simulink model "Predefined_with_GroundTruth_mod22vig1"  (R2022b)
settings: Solver=ode45  StartTime=0.0  StopTime=inf  MaxStep=0.01  RelTol=1e-3
PreLoadFcn:
  | old_index = 1;
model workspace (MAT data in the model file):
  firstWarning = 1
  originalScenarioChecksum = '114339432DE22364D47BB28FC96DC10C'
undefined symbols (not defined in the file or in its folder): Acceleration, ActorID, AngularVelocity, curvature, curvatureAhd, DefaultGear, DEND_B, DEND_S, DEND_T, direction, DiscIntNeverNeededParam, driving, gradbp, L, LF, LR, matlabshared, MAX_BRAKE, MAX_STEER, MAX_TORQUE, MCAR, MIN_BRAKE, MIN_STEER, MIN_TORQUE, NUMD_B, NUMD_S, NUMD_T, Pitch, Position, psi_o, R, Roll, RRdamp, SceneInfo, session, sigbuilder_block, STEER_RATIO, stopSign_ID, Tdead, thetaRefs, TL_ID, TrackWidth, Ts, ts, Vdead, Velocity, WB, X_o, xRef2, xRef2s, Y_o, Yaw, yRef2, yRef2s
libraries: mpcsigdimcheck_private x10, drivingscenarioandsensors x8, drivingvehiclecontroller x2, eeGeneralControl x2, slpidlib x2, simulink x2, trackingutilitieslib x2, mpclib x1, mpcadaslib x1, robotalgslib x1, simulink_extras x1, drivinglib x1
(part 1 of 3)
settings Model: Creator=akshran  LastModifiedBy=rahulmathias
settings DataIOCC: SignalLogging=off
settings DebuggingCC: UnconnectedInputMsg=warning  UnconnectedOutputMsg=warning  UnconnectedLineMsg=warning
settings HardwareCC: ProdBitPerLong=64  ProdHWDeviceType=Intel->x86-64 (Mac OS X)
settings ModelReferenceCC: EnableRefExpFcnMdlSchedulingChecks=on
settings RTWCC: DLArmComputeVersion=19.05

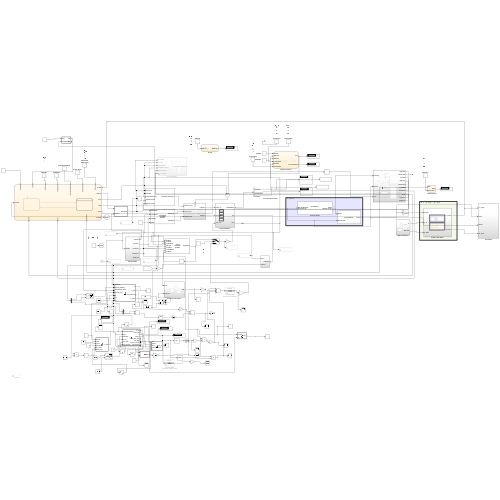
[thumbnail: Simulink's stored preview of the top-level diagram]
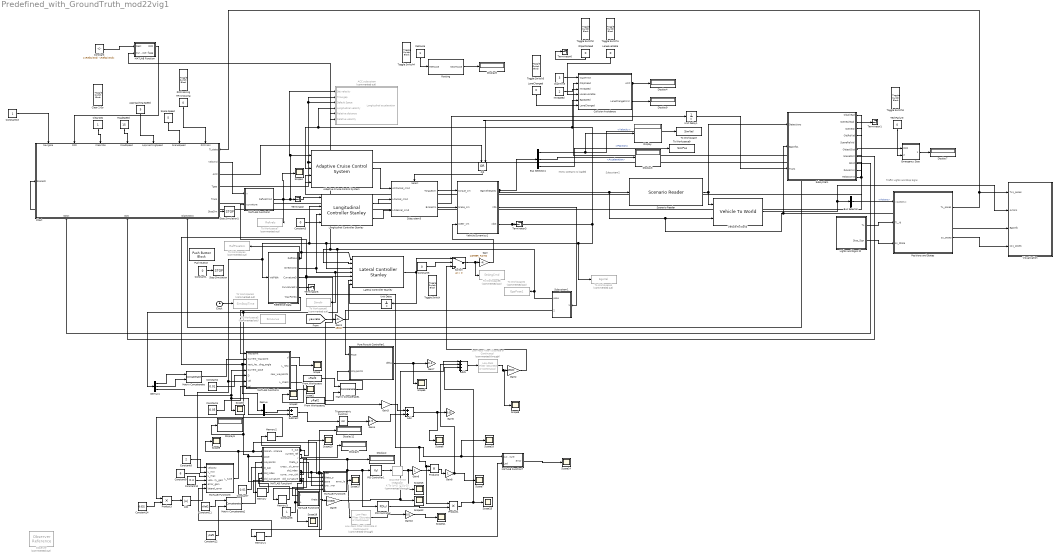
== system Predefined_with_GroundTruth_mod22vig1 ==
  note: Subsystem2
  note: Mcity scenario is loaded
  note: Traffic Lights and Stop Signs
  ACC subsystem : Subsystem  Commented=on
  Abs : Abs  SaturateOnIntegerOverflow=off
  Adaptive Cruise Control System : mpcadaslib/Adaptive Cruise Control System  EgoModel=tf(1,[0.5,1,0])  InitialEgoVelocity=0  DefaultSpacing=WB+2  MaxVelocity=50  MinAcceleration=-40  amin_ext=off  MaxAcceleration=40  amax_ext=off  Ts=0.1  PredictionHorizon=10  ControllerBehavior=1.0  suboptimal=off  maxiter=10  datatypeopt=double  optmode=off  trackmode=off
  Add : Sum
  Add1 : Sum  Inputs=++++
  Approaching Speed : Constant  Value=5
  Bus Selector : BusSelector  OutputSignals=Actors
  Bus Selector4 : BusSelector  OutputSignals=Velocity,Acceleration,Position
  Chart : Stateflow chart  TreatAsAtomicUnit=on
      settings: PortSchema="{\"entries\":[{\"content\":{\"sides\":[{\"content\":{\"connectorIds\":[\"In12\"]},\"type\":\"ConnectorPlacement.EquallySpacedRectSide\",\"uuid\":\"81aca70f-0947-49fb-b60a-be241e44193b\"},{\"content\":{\"connectorIds\":[\"In1\",\"Out1\",\"Out2\",\"Out3\",\"Out4\",\"Out5\"],\"side\":\"RIGHT\"},\"type\":\"ConnectorPlacement.EquallySpacedRectSide\",\"uuid\":\"e7b9645e-3711-4964-ac9b-0199dd335e99\"},{\"content\":{\"connectorIds\":[\"In8\",\"In9\",\"In10\",\"In11\",\"In2\",\"In4\",\"In6\"],\"side\":\"TOP\"},\"type\":\"ConnectorPlacement.EquallySpacedRectSide\",\"uuid\":\"6876f024-944b-4540-9404-d68f37763657\"},{\"content\":{\"connectorIds\":[\"In5\",\"In7\",\"In3\"],\"side\":\"BOTTOM\"},\"type\":\"ConnectorPlacement.EquallySpacedRectSide\",\"uuid\":\"44acab73-cdde-4edf-95df-27422644ccab\"}]},\"type\":\"ConnectorPlacement.EquallySpacedConnector\",\"uuid\":\"d2c31c01-e447-43db-8d2b-8b98a0ca291a\"}],\"packageUris\":[\"http://schema.mathworks.com/mf0/Connector/R2020b\"],\"version\":\"1.0\"}"
  Clear 2 Go : ToggleSwitchBlock
      settings: Values={{'Off', 'On'}, [0 1]}
  Clear2Go : Constant
  Clock : Clock
  Collision Avoidance : Stateflow chart  TreatAsAtomicUnit=on
  Constant : Constant  Value=[xRef2s(end) -yRef2s(end)]
  Constant1 : Constant  Value=0
  Constant10 : Constant  Value=0.4
  Constant11 : Constant  Value=xRef2
  Constant12 : Constant  Value=yRef2
  Constant13 : Constant
  Constant14 : Constant  Value=0.032
  Constant2 : Constant  Value=0.01
  Constant3 : Constant  Value=0
  Constant4 : Constant  Value=0.05
  Constant5 : Constant  Value=0
  Constant6 : Constant  Value=L
  Constant7 : Constant  Value=0.01
  Constant8 : Constant  Value=2
  Constant9 : Constant  Value=6
  Demux : Demux  Outputs=3
  Demux1 : Demux  Outputs=3
  Discrete-Time Integrator : DiscreteIntegrator  Commented=through  IntegratorMethod=Integration: Trapezoidal  SampleTime=-1  ICPrevOutput=DiscIntNeverNeededParam  ICPrevScaledInput=DiscIntNeverNeededParam
  Display{,2..9,12} (10 alike) : Display
  Emergency Stop : Stateflow chart  TreatAsAtomicUnit=on
  From Workspace : FromWorkspace  VariableName=xRef2
  From Workspace1 : FromWorkspace  VariableName=yRef2
  Gain : Gain  Gain=1/STEER_RATIO
  Gain1 : Gain  Gain=180/pi
  Gain10 : Gain  Gain=0.01
  Gain2 : Gain  Gain=180/pi
  Gain3 : Gain  Gain=6*6/2
  Gain4 : Gain  Gain=3.5
  Gain5 : Gain  Gain=0.05
  Gain6 : Gain
  Gain7 : Gain  Gain=0.4
  Gain8 : Gain
  Gain9 : Gain  Gain=0.5305
  LaneAvailable : Constant  Value=0
  LaneChanged : Constant  Value=0
  Lateral Controller Stanley : drivingvehiclecontroller/Lateral Controller Stanley  ModelType=Dynamic bicycle model  PositionGainF=2.5  PositionGainR=2.5  YawRateGain=0.2  DelayGain=0.2  VehicleMass=MCAR  Lf=LF  Lr=LR  TireStiffness=5e3  Wheelbase=3  MaxSteeringAngle=80
  Lights and Signs ID : Subsystem
  Longitudinal Controller Stanley : drivingvehiclecontroller/Longitudinal Controller Stanley  Kp=10  Ki=0.1  SampleTime=0.05  MaxAcceleration=40  MaxDeceleration=40
  Low-Pass Filter (Discrete or Continuous) : eeGeneralControl/Low-Pass Filter (Discrete or Continuous)  Commented=through  K=1  T=0.5  B=inf  A=-inf  init_option=Inherited from block input  x0=0  Ts=-1
  Low-Pass Filter (Discrete or Continuous)2 : eeGeneralControl/Low-Pass Filter (Discrete or Continuous)  Commented=through  K=1  T=1.2  B=inf  A=-inf  init_option=Inherited from block input  x0=0  Ts=-1
  MATLAB Function : MATLAB Function  TreatAsAtomicUnit=on
  MATLAB Function1 : MATLAB Function  TreatAsAtomicUnit=on
  MATLAB Function2 : MATLAB Function  TreatAsAtomicUnit=on
  MATLAB Function3 : MATLAB Function  TreatAsAtomicUnit=on
  MATLAB Function4 : MATLAB Function  TreatAsAtomicUnit=on
  MATLAB Function5 : MATLAB Function  TreatAsAtomicUnit=on
  MATLAB Function6 : MATLAB Function  TreatAsAtomicUnit=on
  MATLAB Function7 : MATLAB Function  TreatAsAtomicUnit=on
  Matrix Concatenate : Concatenate  Mode=Multidimensional array  ConcatenateDimension=2
  Matrix Concatenate1 : Concatenate  Mode=Multidimensional array  ConcatenateDimension=2
  Matrix Concatenate2 : Concatenate  Mode=Multidimensional array  ConcatenateDimension=2
  Memory : Memory  InitialCondition=1  LinearizeMemory=on
  Memory1 : Memory  LinearizeMemory=on
  Memory2 : Memory  LinearizeMemory=on
  Memory3 : Memory  LinearizeMemory=on
  MinSpeed : Constant  Value=2
  OR : Logic  Operator=OR  IconShape=distinctive  AllPortsSameDT=off  OutDataTypeStr=fixdt(1,16)
  ObjectAhead : Constant  Value=0
  Observer : ObserverReference  Commented=on  ObserverModelName=Predefined_with_GroundTruth_mod22_Observer1
  PID Controller : slpidlib/PID Controller  Controller=PD  Form=Parallel  TimeDomain=Discrete-time  UseExternalTs=off  SampleTime=-1  IntegratorMethod=Forward Euler  FilterMethod=Forward Euler  ControllerParametersSource=internal  P=0.0  I=1  UseKiTs=off  D=0.4616  N=100  UseFilter=on  TunerSelectOption=Transfer Function Based (PID Tuner App)  InitialConditionSource=internal  InitialConditionForIntegrator=0  InitialConditionForFilter=0  DifferentiatorICPrevScaledInput=0  ExternalReset=none  TrackingMode=off  Kt=1  LimitOutput=off  SatLimitsSource=internal  UpperSaturationLimit=inf  LowerSaturationLimit=-inf  LinearizeAsGain=on  AntiWindupMode=none  Kb=1  LimitIntegrator=off  UpperIntegratorSaturationLimit=inf  LowerIntegratorSaturationLimit=-inf  POutMin=[]  POutMax=[]  IOutMin=[]  IOutMax=[]  DOutMin=[]  DOutMax=[]  NOutMin=[]  NOutMax=[]  SumOutMin=[]  SumOutMax=[]  SaturationOutMin=[]  SaturationOutMax=[]  PParamMin=[]  PParamMax=[]  IParamMin=[]  IParamMax=[]  DParamMin=[]  DParamMax=[]  NParamMin=[]  NParamMax=[]  KbParamMin=[]  KbParamMax=[]  KtParamMin=[]  KtParamMax=[]  KbOutMin=[]  KbOutMax=[]  KtOutMin=[]  KtOutMax=[]  IntegratorOutMin=[]  IntegratorOutMax=[]  FilterOutMin=[]  FilterOutMax=[]  SumI1OutMin=[]  SumI1OutMax=[]  SumI2OutMin=[]  SumI2OutMax=[]  SumI3OutMin=[]  SumI3OutMax=[]  SumI4OutMin=[]  SumI4OutMax=[]  SumDOutMin=[]  SumDOutMax=[]  DifferentiatorOutMin=[]  DifferentiatorOutMax=[]  FilterDiffOutCoefMin=[]  FilterDiffOutCoefMax=[]  ReciprocalOutMin=[]  ReciprocalOutMax=[]  SumDenOutMin=[]  SumDenOutMax=[]  SumNumOutMin=[]  SumNumOutMax=[]  DivideOutMin=[]  DivideOutMax=[]  UdiffTsProdOutMin=[]  UdiffTsProdOutMax=[]  NTsProdOutMin=[]  NTsProdOutMax=[]  UintegralTsProdOutMin=[]  UintegralTsProdOutMax=[]  UngainTsProdOutMin=[]  UngainTsProdOutMax=[]  ClampingZeroOutDataTypeStr=Inherit: Inherit via back propagation  ClampingZeroOutMin=[]  ClampingZeroOutMax=[]  FilterDenConstantOutDataTypeStr=Inherit: Inherit via back propagation  FilterDenConstantOutMin=[]  FilterDenConstantOutMax=[]  PCopyOutDataTypeStr=Inherit: Inherit via back propagation  PCopyOutMin=[]  PCopyOutMax=[]  NCopyOutDataTypeStr=Inherit: Inherit via back propagation  NCopyOutMin=[]  NCopyOutMax=[]  IntegratorContinuousStateAttributes=''  IntegratorStateMustResolveToSignalObject=off  IntegratorRTWStateStorageClass=Auto  FilterContinuousStateAttributes=''  FilterStateMustResolveToSignalObject=off  FilterRTWStateStorageClass=Auto  ParallelPVariant=InternalParameters  IdealPVariant=Disabled  IVariant=Disabled  DVariant=InternalParameters  IntegratorVariant=Disabled  SatVariant=Disabled  AWVariant=Disabled  PCopyVariant=Disabled  TRVariant=Disabled  FdbkBlocksVariant=Forward  IdealPFdbkVariant=Disabled  SatFdbkVariant=Disabled  DerivativeFilterVariant=ForwardEulerFilter  NVariant=InternalParameters  NCopyVariant=Disabled  FilterICVariant=InternalICsFilter  IntegratorICVariant=Disabled  ExternalResetVariant=Disabled  TRSumVariant=Passthrough  SumFdbkVariant=Disabled  SumVariant=Sum_PD  TsampFilterVariant=InternalTs  TsampNgainVariant=Passthrough  TsampIntegralVariant=Disabled_SignalSpec  ExternalSaturationOutDataTypeStr=Inherit: Same as second input
  PID Controller1 : slpidlib/PID Controller  Controller=I  Form=Parallel  TimeDomain=Discrete-time  UseExternalTs=off  SampleTime=-1  IntegratorMethod=Trapezoidal  FilterMethod=Forward Euler  ControllerParametersSource=internal  P=1  I=0.0079  UseKiTs=on  D=0  N=100  UseFilter=on  TunerSelectOption=Transfer Function Based (PID Tuner App)  InitialConditionSource=internal  InitialConditionForIntegrator=0  InitialConditionForFilter=0  DifferentiatorICPrevScaledInput=0  ExternalReset=none  TrackingMode=off  Kt=1  LimitOutput=off  SatLimitsSource=internal  UpperSaturationLimit=inf  LowerSaturationLimit=-inf  LinearizeAsGain=on  AntiWindupMode=none  Kb=1  LimitIntegrator=off  UpperIntegratorSaturationLimit=inf  LowerIntegratorSaturationLimit=-inf  POutMin=[]  POutMax=[]  IOutMin=[]  IOutMax=[]  DOutMin=[]  DOutMax=[]  NOutMin=[]  NOutMax=[]  SumOutMin=[]  SumOutMax=[]  SaturationOutMin=[]  SaturationOutMax=[]  PParamMin=[]  PParamMax=[]  IParamMin=[]  IParamMax=[]  DParamMin=[]  DParamMax=[]  NParamMin=[]  NParamMax=[]  KbParamMin=[]  KbParamMax=[]  KtParamMin=[]  KtParamMax=[]  KbOutMin=[]  KbOutMax=[]  KtOutMin=[]  KtOutMax=[]  IntegratorOutMin=[]  IntegratorOutMax=[]  FilterOutMin=[]  FilterOutMax=[]  SumI1OutMin=[]  SumI1OutMax=[]  SumI2OutMin=[]  SumI2OutMax=[]  SumI3OutMin=[]  SumI3OutMax=[]  SumI4OutMin=[]  SumI4OutMax=[]  SumDOutMin=[]  SumDOutMax=[]  DifferentiatorOutMin=[]  DifferentiatorOutMax=[]  FilterDiffOutCoefMin=[]  FilterDiffOutCoefMax=[]  ReciprocalOutMin=[]  ReciprocalOutMax=[]  SumDenOutMin=[]  SumDenOutMax=[]  SumNumOutMin=[]  SumNumOutMax=[]  DivideOutMin=[]  DivideOutMax=[]  UdiffTsProdOutMin=[]  UdiffTsProdOutMax=[]  NTsProdOutMin=[]  NTsProdOutMax=[]  UintegralTsProdOutMin=[]  UintegralTsProdOutMax=[]  UngainTsProdOutMin=[]  UngainTsProdOutMax=[]  ClampingZeroOutDataTypeStr=Inherit: Inherit via back propagation  ClampingZeroOutMin=[]  ClampingZeroOutMax=[]  FilterDenConstantOutDataTypeStr=Inherit: Inherit via back propagation  FilterDenConstantOutMin=[]  FilterDenConstantOutMax=[]  PCopyOutDataTypeStr=Inherit: Inherit via back propagation  PCopyOutMin=[]  PCopyOutMax=[]  NCopyOutDataTypeStr=Inherit: Inherit via back propagation  NCopyOutMin=[]  NCopyOutMax=[]  IntegratorContinuousStateAttributes=''  IntegratorStateMustResolveToSignalObject=off  IntegratorRTWStateStorageClass=Auto  FilterContinuousStateAttributes=''  FilterStateMustResolveToSignalObject=off  FilterRTWStateStorageClass=Auto  ParallelPVariant=Disabled  IdealPVariant=Disabled  IVariant=InternalParameters  DVariant=Disabled  IntegratorVariant=Discrete  SatVariant=Disabled  AWVariant=Passthrough  PCopyVariant=Disabled  TRVariant=Disabled  FdbkBlocksVariant=Forward  IdealPFdbkVariant=Disabled  SatFdbkVariant=Disabled  DerivativeFilterVariant=Disabled  NVariant=Disabled  NCopyVariant=Disabled_SignalSpec  FilterICVariant=Disabled  IntegratorICVariant=InternalICs  ExternalResetVariant=Disabled  TRSumVariant=Passthrough  SumFdbkVariant=Disabled  SumVariant=Passthrough_I  TsampFilterVariant=InternalTs  TsampNgainVariant=Passthrough  TsampIntegralVariant=Passthrough  ExternalSaturationOutDataTypeStr=Inherit: Same as second input
  "Positions and States " : Subsystem
  Product1 : Product
  Product2 : Product
  Product3 : Product
  Pure Pursuit Controller1 : Subsystem
  Push Button : PushButtonBlock  OffValue=0.000000
  RR Crossing : Constant  Value=0
  RRCrossing : ToggleSwitchBlock
      settings: Values={{'Off', 'On'}, [0 1]}
  ReRoute : Constant
  Reference Data : Subsystem  VariantControl=Stanley
  RoadSpeed : Constant  Value=15
  Routing : Stateflow chart  TreatAsAtomicUnit=on
  Scenario Reader : drivingscenarioandsensors/Scenario Reader  ScenarioSource=From file  ScenarioFileName=/Users/vigneshsrinivasan/Downloads/ad2_y1_simulationpkg/scenarios/Roundabout.mat  ScenarioVariableName=scenario  OutputCoordinateSystem=Vehicle coordinates  EgoVehicleSource=Input port  EgoVehicleActorID=1  OrientVehiclesOnRoad=on  OutputEgoVehiclePose=on  OutputEgoVehicleState=off  SampleTime=Ts  LaneBoundaryOutput=None  LaneBoundaryDistance=0:0.5:9.5  LaneBoundaryLocation=Center of lane markings  BusNameSource=Auto  BusName=BusActors  BusNumActorsSource=Scenario  BusNumActors=100  BusName2Source=Auto  BusName2=BusLaneBoundaries  BusNumLaneBoundariesSource=Scenario  BusNumLaneBoundaries=10  BusName3Source=Auto  BusName3=BusEgoActor  BusName4Source=Auto  BusName4=BusEgoState  ShowCoordinateLabels=on  SimulateUsing=Interpreted execution
  Scene Speed : Constant  Value=5
  Scope{,1..15,17..19} (19 alike) : Scope
  Stop Simulation : Stop
  Stop Simulation1 : Stop
  Subsystem : Subsystem
  Subsystem1 : Subsystem
  Subsystem3 : Subsystem
      settings: PortSchema="{\"entries\":[{\"content\":{\"sides\":[{\"content\":{\"connectorIds\":[\"In1\",\"In2\",\"In3\"]},\"type\":\"ConnectorPlacement.EquallySpacedRectSide\",\"uuid\":\"a23b1a10-3bcb-40a0-900c-c9a3f160b173\"},{\"content\":{\"connectorIds\":[\"Out1\",\"Out2\"],\"side\":\"RIGHT\"},\"type\":\"ConnectorPlacement.EquallySpacedRectSide\",\"uuid\":\"88840b66-912f-4184-aeec-297642319416\"},{\"content\":{\"connectorIds\":[\"In4\"],\"side\":\"TOP\"},\"type\":\"ConnectorPlacement.EquallySpacedRectSide\",\"uuid\":\"37a03ca9-b065-473e-b290-3b07703c6005\"}]},\"type\":\"ConnectorPlacement.EquallySpacedConnector\",\"uuid\":\"5bfc7c71-8f7a-4cba-a168-7eeca22a2fcb\"}],\"packageUris\":[\"http://schema.mathworks.com/mf0/Connector/R2020b\"],\"version\":\"1.0\"}"
  Subtract : Sum  Inputs=+-
  Switch : Switch  Criteria=u2 > Threshold  SaturateOnIntegerOverflow=off  InputSameDT=off
  TechFailure : Constant  Value=0
  Terminator{,1,3,5..6} (5 alike) : Terminator
  To Workspace : ToWorkspace  VariableName=SimVel  SampleTime=-1
      settings: Save2DSignal=2-D array (concatenate along first dimension)
  To Workspace1 : ToWorkspace  Commented=on  VariableName=EgoVel  SampleTime=-1
      settings: Save2DSignal=2-D array (concatenate along first dimension)
  To Workspace2 : ToWorkspace  Commented=on  VariableName=EgoPose1  SampleTime=-1
      settings: Save2DSignal=2-D array (concatenate along first dimension)
  To Workspace3 : ToWorkspace  Commented=on  VariableName=SimStopTime  SampleTime=-1
      settings: Save2DSignal=2-D array (concatenate along first dimension)
  To Workspace4 : ToWorkspace  Commented=on  VariableName=RefPoseSim  SampleTime=-1
      settings: Save2DSignal=2-D array (concatenate along first dimension)
  To Workspace5 : ToWorkspace  Commented=on  VariableName=Simcurve  SaveFormat=Timeseries  SampleTime=-1
      settings: Save2DSignal=2-D array (concatenate along first dimension)
  To Workspace6 : ToWorkspace  Commented=on  VariableName=Simdir  SaveFormat=Timeseries  SampleTime=-1
      settings: Save2DSignal=2-D array (concatenate along first dimension)
  To Workspace7 : ToWorkspace  Commented=on  VariableName=Refvels  SaveFormat=Timeseries  SampleTime=-1
      settings: Save2DSignal=2-D array (concatenate along first dimension)
  To Workspace8 : ToWorkspace  Commented=on  VariableName=StrAngCmd  SampleTime=-1
      settings: Save2DSignal=2-D array (concatenate along first dimension)
  To Workspace9 : ToWorkspace  VariableName=SimPos  SampleTime=-1
      settings: Save2DSignal=2-D array (concatenate along first dimension)
  Toggle Switch{,1..5} (6 alike) : ToggleSwitchBlock
      settings: Values={{'Off', 'On'}, [0 1]}
  Trigonometric Function : Trigonometry
  Unit Delay : UnitDelay  SampleTime=-1  HasFrameUpgradeWarning=on
  Unit Delay1 : UnitDelay  SampleTime=-1  HasFrameUpgradeWarning=on
  Vehicle Dynamics1 : Subsystem
  Vehicle To World : drivingscenarioandsensors/Vehicle To World  BusNameSource=Auto  BusName=BusVehicleToWorldActors  SimulateUsing=Interpreted execution
  Visualization : Subsystem
  WaitTime : Constant  Value=3
  wires:
  "Positions and States "/1(TL_poses) -> Chart/1(TLstate), Visualization/1(TL1_poses)
  "Positions and States "/2(ss_poses) -> Visualization/4(ss1_poses)
  Lights and Signs ID/2(Stop_Sign) -> "Positions and States "/3(ss_State)
  Bus Selector/1 -> "Positions and States "/1(<Actors>)  "<Actors>"
  Lights and Signs ID/1(TL) -> "Positions and States "/2(TL_id)
  Unit Delay/1 -> Lateral Controller Stanley/7
  Lateral Controller Stanley/1 -> Switch/1, Unit Delay/1
  Vehicle Dynamics1/2(Info) -> Subsystem1/1(VehFdbk)
  Constant3/1 -> Longitudinal Controller Stanley/4
  Bus Selector4/1 -> Display/1, To Workspace/1  "<Velocity>"
  Bus Selector4/2 -> Display3/1  "<Acceleration>"
  Vehicle Dynamics1/3(xdot) -> To Workspace1/1, Longitudinal Controller Stanley/2, MATLAB Function1/6(vel), MATLAB Function3/1(velocity), Reference Data/1(VelFdbk), Lateral Controller Stanley/3, Collision Avoidance/5(EgoSpeed), ACC subsystem/4(Longitudinal velocity), Adaptive Cruise Control System/3, Terminator3/1
  Reference Data/2(DirectionO) -> To Workspace6/1, Lateral Controller Stanley/4, Longitudinal Controller Stanley/3
  [yawrate] -> Gain1/1
  Gain1/1 -> Lateral Controller Stanley/6
  Approaching Speed/1 -> Chart/2(ApproachingSpeed)
  Scene Speed/1 -> Chart/4(SceneSpeed)
  Gain/1 -> Vehicle Dynamics1/3(steer_cm)
  RR Crossing/1 -> Chart/6(RRCross)
  Clear2Go/1 -> Chart/10(Clear2Go)
  RoadSpeed/1 -> Chart/11(RoadSpeed)
  TechFailure/1 -> Emergency Stop/2(TechFailure)
  Emergency Stop/1(EStop) -> Display7/1
  Collision Avoidance/1(ACC) -> OR/2, Display4/1
  MinSpeed/1 -> Collision Avoidance/3(MinSpeed)
  WaitTime/1 -> Collision Avoidance/1(WaitTime)
  LaneAvailable/1 -> Collision Avoidance/4(LaneAvailable)
  ReRoute/1 -> Routing/1(ReRoute)
  Routing/1(NewRoute) -> Display8/1
  Chart/3(Tgap) -> ACC subsystem/3(Default Space), ACC subsystem/2(Time gap), Adaptive Cruise Control System/2
  LaneChanged/1 -> Collision Avoidance/6(LaneChanged)
  Collision Avoidance/2(LaneChangeCmd) -> Display9/1
  Longitudinal Controller Stanley/1 -> Subsystem3/2(LCaccel_cmd)
  Longitudinal Controller Stanley/2 -> Subsystem3/3(LCdeccel_cmd)
  Subsystem3/1(TorgueCm) -> Vehicle Dynamics1/1(torque_cm)
  Subsystem3/2(BrakeCm) -> Vehicle Dynamics1/2(brake_cm)
  MATLAB Function2/1(RefVelCmd) -> Scope4/1, To Workspace7/1, Adaptive Cruise Control System/1, ACC subsystem/1(Set velocity), Longitudinal Controller Stanley/1, Terminator/1
  Clock/1 -> To Workspace3/1
  Reference Data/4(CurvatureO1) -> Terminator5/1
  Subsystem1/2(PPpose) -> Pure Pursuit Controller1/1(Pose)
  Constant5/1 -> Switch/2
  Switch/1 -> To Workspace8/1, Gain/1
  Chart/1(VelCmd) -> MATLAB Function2/1(v)
  Subsystem/6(ObjectDist) -> Chart/3(ObjectDist), Emergency Stop/1(D2O)
  Subsystem/4(ObjRelVel) -> Adaptive Cruise Control System/5
  Subsystem/1(ObjAhead) -> Collision Avoidance/2(ObjAhead)
  Subsystem/2(SceneAhead) -> Terminator1/1
  Subsystem/3(SceneID) -> Chart/12(SceneID)
  Subsystem/8(SDist) -> Chart/5(SDist)
  Subsystem/7(SceneDist) -> Chart/7(D2S)
  Vehicle To World/1 -> Visualization/2(Actors), Bus Selector/1
  Scenario Reader/1 -> Subsystem/1(Detections), Vehicle To World/1
  Vehicle Dynamics1/1(EgoVehStates) -> Visualization/3(EgoInfo), Subsystem/2(EgoInfo1), Vehicle To World/2, Scenario Reader/1, Bus Selector4/1
  OR/1 -> Subsystem3/4(Select)
  Chart/2(ACC) -> OR/1
  Subsystem/9(ReVelmin) -> ACC subsystem/6(Relative velocity)
  Subsystem/10(RelDistmin) -> Adaptive Cruise Control System/4, ACC subsystem/5(Relative distance)
  Chart/4(Trans) -> Unit Delay1/1
  Unit Delay1/1 -> Subsystem/3(Trans)
  Adaptive Cruise Control System/1 -> Subsystem3/1(ACCaccel_cmd)
  Constant/1 -> MATLAB Function/1(Dest)
  MATLAB Function/1(D2D) -> Chart/9(D2D)
  Chart/5(StopSim) -> Stop Simulation1/1
  Bus Selector4/3 -> To Workspace9/1  "<Position>"
  Constant1/1 -> Stop Simulation/1
  Reference Data/5(WayPoints) -> MATLAB Function1/1(Waypoint)
  Subsystem1/1(pose) -> To Workspace2/1, Demux1/1, MATLAB Function4/2(pose), MATLAB Function5/3(pose), Display6/1, Lateral Controller Stanley/2, MATLAB Function/2(CurrentPose)
  Constant2/1 -> MATLAB Function1/5(D)
  MATLAB Function1/1(d) -> Scope/1
  MATLAB Function1/2(L_new) -> Scope1/1
  ObjectAhead/1 -> Terminator6/1
  Demux1/3 -> Scope3/1, Subtract/2, MATLAB Function1/4(Current_pose)
  Demux1/2 -> Matrix Concatenate/2
  Demux1/1 -> Matrix Concatenate/1
  Reference Data/1(RefPose) -> To Workspace4/1, Demux/1, MATLAB Function1/3(next_heading_angle), Lateral Controller Stanley/1
  Matrix Concatenate/1 -> MATLAB Function1/2(Current_Waypoint)
  MATLAB Function1/4(L_check) -> Scope2/1
  Constant4/1 -> MATLAB Function1/7(tol)
  Trigonometric Function/1 -> Gain4/1
  Add/1 -> Scope6/1, Gain5/1
  Demux/3 -> Subtract/1
  Subtract/1 -> Trigonometric Function/1
  Gain3/1 -> Add/1
  Gain4/1 -> Add/2
  Pure Pursuit Controller1/1(delta) -> Scope5/1, Gain7/1
  Discrete-Time Integrator/1 -> Scope15/1, Gain6/1
  Add1/1 -> Low-Pass Filter (Discrete or Continuous)/1
  Low-Pass Filter (Discrete or Continuous)/1 -> Scope8/1, Gain2/1
  Gain8/1 -> Add1/2, Scope7/1
  From Workspace1/1 -> Matrix Concatenate1/2
  From Workspace/1 -> Matrix Concatenate1/1
  Matrix Concatenate1/1 -> Pure Pursuit Controller1/2(Waypoints)
  MATLAB Function3/1(L_tune) -> Scope9/1, MATLAB Function7/2(Lad), MATLAB Function5/1(Lad), MATLAB Function4/1(lookahead_distance)
  Constant11/1 -> Matrix Concatenate2/1
  Constant12/1 -> Matrix Concatenate2/2
  Matrix Concatenate2/1 -> MATLAB Function4/3(waypoints)
  Constant7/1 -> MATLAB Function4/4(D_sat)
  Constant8/1 -> MATLAB Function3/2(L_min)
  Constant9/1 -> MATLAB Function3/3(L_max)
  Constant10/1 -> MATLAB Function3/4(velocity_gain)
  MATLAB Function5/1(error_la) -> Low-Pass Filter (Discrete or Continuous)2/1
  Gain2/1 -> Switch/3
  Constant6/1 -> MATLAB Function5/5(L), MATLAB Function6/2(L)
  MATLAB Function4/3(r) -> MATLAB Function6/1(r)
  Low-Pass Filter (Discrete or Continuous)2/1 -> Gain10/1
  Gain10/1 -> Scope11/1
  MATLAB Function4/2(current_ref) -> Display5/1
  Gain9/1 -> Scope12/1, Add1/1
  Memory/1 -> MATLAB Function4/5("old_index ")
  Constant13/1 -> Chart/8(Navigate)
  PID Controller1/1 -> Discrete-Time Integrator/1
  MATLAB Function6/1(theta) -> Gain9/1
  MATLAB Function7/1(error) -> Scope14/1
  MATLAB Function4/1(K_out) -> Memory2/1, Scope10/1
  MATLAB Function4/7(current_error_chk) -> Display2/1, Scope17/1, PID Controller/1, PID Controller1/1
  PID Controller/1 -> Product1/2
  Product1/1 -> Add1/3, Scope13/1
  Gain6/1 -> Product2/2
  Product2/1 -> Gain8/1
  MATLAB Function4/6(old_index) -> Scope19/1, Memory/1, Memory1/1, Display12/1, MATLAB Function5/4(cross_track_error)
  Memory1/1 -> MATLAB Function3/6(lateral_error)
  Constant14/1 -> Product3/2
  Product3/1 -> Abs/1
  Abs/1 -> MATLAB Function3/5(error_gain)
  MATLAB Function4/4(theta_p) -> MATLAB Function5/2(theta_p)
  MATLAB Function4/8(old_curvature) -> Memory3/1
  Memory3/1 -> MATLAB Function4/6("old_curvature ")
  Memory2/1 -> Product3/1
  Reference Data/3(CurvatureO) -> Product1/1, Product2/1, Scope18/1, MATLAB Function7/1(curvature), MATLAB Function2/2(curvature), Lateral Controller Stanley/5, Gain3/1

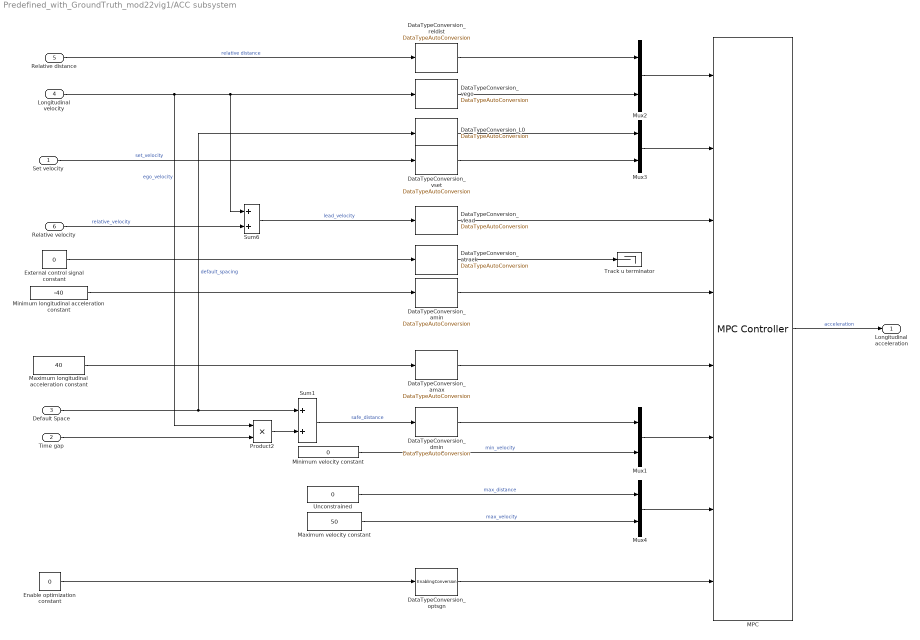
== system Predefined_with_GroundTruth_mod22vig1/ACC subsystem ==
  Set velocity : Inport
  Time gap : Inport  Port=2
  Default Space : Inport  Port=3
  Longitudinal velocity : Inport  Port=4
  Relative distance : Inport  Port=5
  Relative velocity : Inport  Port=6
  DataTypeConversion_L0 : mpcsigdimcheck_private/DataTypeAutoConversion  datatypestr=accsubsystem_data.DataType
  DataTypeConversion_amax : mpcsigdimcheck_private/DataTypeAutoConversion  datatypestr=accsubsystem_data.DataType
  DataTypeConversion_amin : mpcsigdimcheck_private/DataTypeAutoConversion  datatypestr=accsubsystem_data.DataType
  DataTypeConversion_atrack : mpcsigdimcheck_private/DataTypeAutoConversion  datatypestr=accsubsystem_data.DataType
  DataTypeConversion_dmin : mpcsigdimcheck_private/DataTypeAutoConversion  datatypestr=accsubsystem_data.DataType
  DataTypeConversion_optsgn : mpcsigdimcheck_private/EnablingConversion  SystemSampleTime=-1  VariantActivationTime=update diagram  Latency=0  AutoFrameSizeCalculation=off
  DataTypeConversion_reldist : mpcsigdimcheck_private/DataTypeAutoConversion  datatypestr=accsubsystem_data.DataType
  DataTypeConversion_vego : mpcsigdimcheck_private/DataTypeAutoConversion  datatypestr=accsubsystem_data.DataType
  DataTypeConversion_vlead : mpcsigdimcheck_private/DataTypeAutoConversion  datatypestr=accsubsystem_data.DataType
  DataTypeConversion_vset : mpcsigdimcheck_private/DataTypeAutoConversion  datatypestr=accsubsystem_data.DataType
  Enable optimization constant : Constant  Value=0  OutDataTypeStr=accsubsystem_data.DataType
  External control signal constant : Constant  Value=0  OutDataTypeStr=accsubsystem_data.DataType
  MPC : mpclib/MPC Controller  SCDEnableBlockLinearizationSpecification=on  mpcobj=accsubsystem_data.Controller  is_multiple=0  enable_value=0  return_u0=off  updateMPCinCallerWorkspace=off  md_inport=on  mv_inport=off  uref_inport=off  return_cost=off  return_mvseq=off  return_qpstatus=off  return_xseq=off  return_state=off  return_ovseq=off  state_inport=off  umin_inport=on  umax_inport=on  ymin_inport=on  ymax_inport=on  cc_inport=off  ywt_inport=off  uwt_inport=off  duwt_inport=off  rhoeps_inport=off  pm_inport=off  MaximumP=10  HorizonChoice=FixedHorizon  n_ts=0.1  n_p=15  n_mv=1  n_md=1  n_ud=0  n_mo=2  n_uo=0  BlockDataType=double  SampleTimeInherited=off  switch_inport=on
  Maximum longitudinal acceleration constant : Constant  Value=40  OutDataTypeStr=accsubsystem_data.DataType
  Maximum velocity constant : Constant  Value=50  OutDataTypeStr=accsubsystem_data.DataType
  Minimum longitudinal acceleration constant : Constant  Value=-40  OutDataTypeStr=accsubsystem_data.DataType
  Minimum velocity constant : Constant  Value=0  OutDataTypeStr=accsubsystem_data.DataType
  Mux{1..4} (4 alike) : Mux  Inputs=[1 1]
  Product2 : Product
  Sum1 : Sum
  Sum6 : Sum
  Track u terminator : Terminator
  Unconstrained : Constant  Value=0  OutDataTypeStr=accsubsystem_data.DataType
  Longitudinal acceleration : Outport  PortDimensions=1  VectorParamsAs1DForOutWhenUnconnected=off
  wires:
  Sum6/1 -> DataTypeConversion_vlead/1  "lead_velocity"
  Default Space/1 -> DataTypeConversion_L0/1, Sum1/1  "default_spacing"
  Mux2/1 -> MPC/1
  Mux3/1 -> MPC/2
  Longitudinal velocity/1 -> Product2/1, DataTypeConversion_vego/1, Sum6/1  "ego_velocity"
  Relative distance/1 -> DataTypeConversion_reldist/1  "relative distance"
  Relative velocity/1 -> Sum6/2  "relative_velocity"
  MPC/1 -> Longitudinal acceleration/1  "acceleration"
  Product2/1 -> Sum1/2
  Minimum velocity constant/1 -> Mux1/2  "min_velocity"
  Sum1/1 -> DataTypeConversion_dmin/1  "safe_distance"
  Mux1/1 -> MPC/6
  DataTypeConversion_amax/1 -> MPC/5
  DataTypeConversion_amin/1 -> MPC/4
  DataTypeConversion_dmin/1 -> Mux1/1
  DataTypeConversion_vlead/1 -> MPC/3
  DataTypeConversion_L0/1 -> Mux3/1
  DataTypeConversion_vset/1 -> Mux3/2
  DataTypeConversion_reldist/1 -> Mux2/1
  DataTypeConversion_vego/1 -> Mux2/2
  Time gap/1 -> Product2/2
  Set velocity/1 -> DataTypeConversion_vset/1  "set_velocity"
  Minimum longitudinal acceleration constant/1 -> DataTypeConversion_amin/1
  Maximum longitudinal acceleration constant/1 -> DataTypeConversion_amax/1
  Mux4/1 -> MPC/7
  Maximum velocity constant/1 -> Mux4/2  "max_velocity"
  Unconstrained/1 -> Mux4/1  "max_distance"
  Enable optimization constant/1 -> DataTypeConversion_optsgn/1
  DataTypeConversion_optsgn/1 -> MPC/8
  External control signal constant/1 -> DataTypeConversion_atrack/1
  DataTypeConversion_atrack/1 -> Track u terminator/1

== system Predefined_with_GroundTruth_mod22vig1/Lights and Signs ID ==
  Constant : Constant  Value=TL_ID
  Constant1 : Constant  Value=stopSign_ID
  TL : Outport
  Stop_Sign : Outport  Port=2
  wires:
  Constant/1 -> TL/1
  Constant1/1 -> Stop_Sign/1

== system Predefined_with_GroundTruth_mod22vig1/Positions and States  ==
  note: Stop Sign positon
  note: Traffic Light Position and State
  <Actors> : Inport
  TL_id : Inport  Port=2
  ss_State : Inport  Port=3
  MATLAB Function1 : MATLAB Function  TreatAsAtomicUnit=on
  MATLAB Function2 : MATLAB Function  TreatAsAtomicUnit=on
  Traffic Light Sensor : Subsystem  mask{TrafficLightSensorModeSelection=Cycle}
      mask prompts: TrafficLightSensorModeSelection "Traffic Light Sensor Mode:"
      mask TypeOptions TrafficLightSensorModeSelection: Steady Green | Steady Red | Cycle
      mask DialogControl DescTextVar Prompt: Simulate a traffic light sensor.
  TL_poses : Outport
  ss_poses : Outport  Port=2
  wires:
  <Actors>/1 -> MATLAB Function2/1(Actors), MATLAB Function1/1(Actors)
  ss_State/1 -> MATLAB Function2/2(ss_State)
  TL_id/1 -> Traffic Light Sensor/1(TL_id)
  Traffic Light Sensor/1(TL_State) -> MATLAB Function1/2(TL_State)  "TL_State"
  MATLAB Function2/1(ss_poses) -> ss_poses/1
  MATLAB Function1/1(TL_poses) -> TL_poses/1

== system Predefined_with_GroundTruth_mod22vig1/Pure Pursuit Controller1 ==
  note: The subsystem implements a Pure Pursuit controller. The "Pure Pursuit" block calculates the target direction and the "Wheel Steering Angle Formulation" block calculates the wheel steering angle.
  Pose : Inport
  Waypoints : Inport  Port=2
  Pure Pursuit : robotalgslib/Pure Pursuit  DesiredLinearVelocity=1  MaxAngularVelocity=1.0  LookaheadDistance=6  TargetDirPort=on  SimulateUsing=Code generation
  Terminator6 : Terminator
  Terminator7 : Terminator
  Wheel Steering Angle Formulation : Subsystem  mask{L=L, ld=6}
      mask prompts: L "Bicycle length"; ld "Lookahead distance"
      mask TypeOptions L: Bicycle length/Value
      mask TypeOptions ld: Lookahead distance/Value
      mask Display:
      | image("GeometryMask.png")
      | port_label('input', 1, 'alpha')
      | port_label('output', 1, 'delta')
  delta : Outport
  wires:
  Wheel Steering Angle Formulation/1(Al) -> delta/1
  Pure Pursuit/3 -> Wheel Steering Angle Formulation/1(alpha)
  Pure Pursuit/2 -> Terminator7/1
  Pose/1 -> Pure Pursuit/1
  Pure Pursuit/1 -> Terminator6/1
  Waypoints/1 -> Pure Pursuit/2

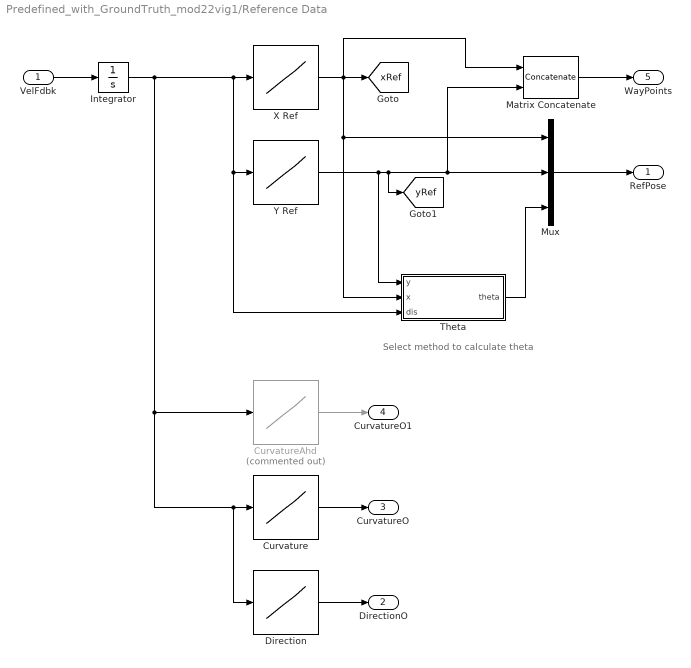
== system Predefined_with_GroundTruth_mod22vig1/Reference Data ==
  note: Select method to calculate theta
  VelFdbk : Inport
  Curvature : Lookup_n-D  NumberOfTableDimensions=1  BreakpointsForDimension1=gradbp  Table=curvature  InternalRulePriority=Speed  RndMeth=Simplest
  CurvatureAhd : Lookup_n-D  Commented=on  NumberOfTableDimensions=1  BreakpointsForDimension1=gradbp  Table=curvatureAhd  InternalRulePriority=Speed  RndMeth=Simplest
  Direction : Lookup_n-D  NumberOfTableDimensions=1  BreakpointsForDimension1=gradbp  Table=direction  InternalRulePriority=Speed  RndMeth=Simplest
  Integrator : Integrator
  Matrix Concatenate : Concatenate  Mode=Multidimensional array  ConcatenateDimension=2
  Mux : Mux  Inputs=3
  Theta : Subsystem  Variant=on  VariantControlMode=label  LabelModeActiveChoice=thetaLookUpTable
  X Ref : Lookup_n-D  NumberOfTableDimensions=1  BreakpointsForDimension1=gradbp  Table=xRef2s  InternalRulePriority=Speed  RndMeth=Simplest
  Y Ref : Lookup_n-D  NumberOfTableDimensions=1  BreakpointsForDimension1=gradbp  Table=yRef2s  InternalRulePriority=Speed  RndMeth=Simplest
  RefPose : Outport
  DirectionO : Outport  Port=2
  CurvatureO : Outport  Port=3
  CurvatureO1 : Outport  Port=4
  WayPoints : Outport  Port=5
  tag scope: xRef=global, yRef=global
  wires:
  Direction/1 -> DirectionO/1
  Curvature/1 -> CurvatureO/1
  Mux/1 -> RefPose/1
  Integrator/1 -> CurvatureAhd/1, Curvature/1, Direction/1, Theta/3(dis), Y Ref/1, X Ref/1
  VelFdbk/1 -> Integrator/1
  Theta/1(theta) -> Mux/3
  CurvatureAhd/1 -> CurvatureO1/1
  Matrix Concatenate/1 -> WayPoints/1
  X Ref/1 -> Theta/2(x), Mux/1, Matrix Concatenate/1, [xRef]
  Y Ref/1 -> Theta/1(y), Matrix Concatenate/2, Mux/2, [yRef]

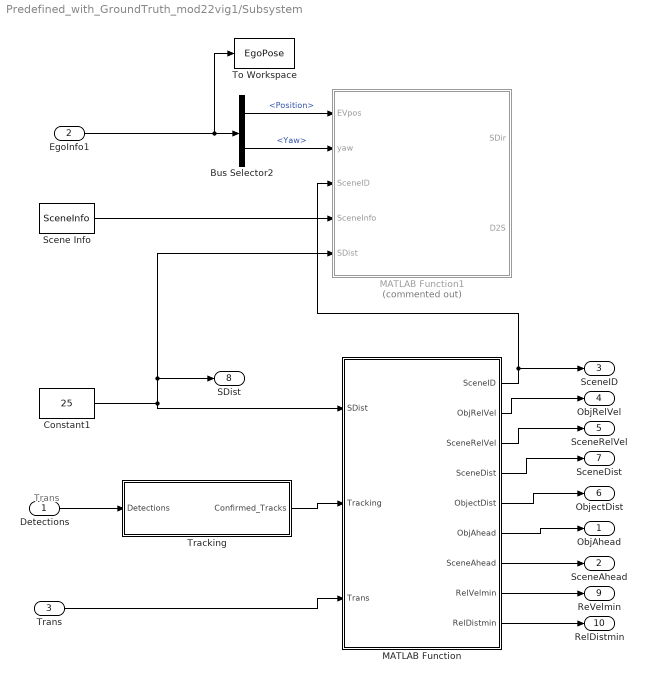
== system Predefined_with_GroundTruth_mod22vig1/Subsystem ==
  note: Trans
  Detections : Inport
  EgoInfo1 : Inport  Port=2
  Trans : Inport  Port=3
  Bus Selector2 : BusSelector  OutputSignals=Position,Yaw
  Constant1 : Constant  Value=25
  MATLAB Function : MATLAB Function  TreatAsAtomicUnit=on
  MATLAB Function1 : MATLAB Function  Commented=on  TreatAsAtomicUnit=on
  Scene Info : Constant  Value=SceneInfo  VectorParams1D=off
  To Workspace : ToWorkspace  VariableName=EgoPose  SaveFormat=Timeseries  SampleTime=-1
  Tracking : Subsystem
  ObjAhead : Outport
  SceneAhead : Outport  Port=2
  SceneID : Outport  Port=3
  ObjRelVel : Outport  Port=4
  SceneRelVel : Outport  Port=5
  ObjectDist : Outport  Port=6
  SceneDist : Outport  Port=7
  SDist : Outport  Port=8
  ReVelmin : Outport  Port=9
  RelDistmin : Outport  Port=10
  wires:
  MATLAB Function/6(ObjAhead) -> ObjAhead/1
  MATLAB Function/5(ObjectDist) -> ObjectDist/1
  MATLAB Function/7(SceneAhead) -> SceneAhead/1
  MATLAB Function/2(ObjRelVel) -> ObjRelVel/1
  EgoInfo1/1 -> To Workspace/1, Bus Selector2/1
  Bus Selector2/1 -> MATLAB Function1/1(EVpos)  "<Position>"
  Detections/1 -> Tracking/1(Detections)
  Scene Info/1 -> MATLAB Function1/4(SceneInfo)
  Bus Selector2/2 -> MATLAB Function1/2(yaw)  "<Yaw>"
  Tracking/1(Confirmed_Tracks) -> MATLAB Function/2(Tracking)
  Constant1/1 -> MATLAB Function1/5(SDist), SDist/1, MATLAB Function/1(SDist)
  MATLAB Function/1(SceneID) -> MATLAB Function1/3(SceneID), SceneID/1
  MATLAB Function/4(SceneDist) -> SceneDist/1
  MATLAB Function/3(SceneRelVel) -> SceneRelVel/1
  MATLAB Function/8(RelVelmin) -> ReVelmin/1
  MATLAB Function/9(RelDistmin) -> RelDistmin/1
  Trans/1 -> MATLAB Function/3(Trans)

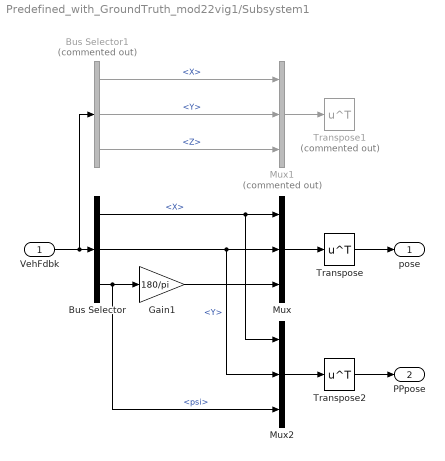
== system Predefined_with_GroundTruth_mod22vig1/Subsystem1 ==
  VehFdbk : Inport
  Bus Selector : BusSelector  OutputSignals=InertFrm.Cg.Disp.X,InertFrm.Cg.Disp.Y,InertFrm.Cg.Ang.psi
  Bus Selector1 : BusSelector  Commented=on  OutputSignals=InertFrm.Cg.Disp.X,InertFrm.Cg.Disp.Y,InertFrm.Cg.Disp.Z
  Gain1 : Gain  Gain=180/pi
  Mux : Mux  Inputs=3
  Mux1 : Mux  Commented=on  Inputs=3
  Mux2 : Mux  Inputs=3
  Transpose : Math  Operator=transpose  SignedPower=on
  Transpose1 : Math  Commented=on  Operator=transpose  SignedPower=on
  Transpose2 : Math  Operator=transpose  SignedPower=on
  pose : Outport
  PPpose : Outport  Port=2
  wires:
  Mux/1 -> Transpose/1
  VehFdbk/1 -> Bus Selector1/1, Bus Selector/1
  Gain1/1 -> Mux/3
  Transpose/1 -> pose/1
  Bus Selector/3 -> Mux2/3, Gain1/1  "<psi>"
  Bus Selector1/1 -> Mux1/1  "<X>"
  Bus Selector1/2 -> Mux1/2  "<Y>"
  Bus Selector1/3 -> Mux1/3  "<Z>"
  Mux1/1 -> Transpose1/1
  Mux2/1 -> Transpose2/1
  Transpose2/1 -> PPpose/1
  Bus Selector/2 -> Mux/2, Mux2/2  "<Y>"
  Bus Selector/1 -> Mux/1, Mux2/1  "<X>"

== system Predefined_with_GroundTruth_mod22vig1/Subsystem3 ==
  ACCaccel_cmd : Inport
  LCaccel_cmd : Inport  Port=2
  LCdeccel_cmd : Inport  Port=3
  Select : Inport  Port=4
  Merge1 : Merge
  Merge2 : Merge
  Subsystem1 : Subsystem
  Subsystem2 : Subsystem
  Switch Case1 : SwitchCase  CaseConditions={1, 0}  ShowDefaultCase=off
  TorgueCm : Outport
  BrakeCm : Outport  Port=2
  wires:
  LCdeccel_cmd/1 -> Subsystem1/2(decc_cmd)
  Subsystem1/2(brake_cm) -> Merge2/2
  Subsystem1/1(torque_cm) -> Merge1/2
  Subsystem2/2(brake_cm) -> Merge2/1
  Switch Case1/1 -> Subsystem2/Action
  Switch Case1/2 -> Subsystem1/Action
  Subsystem2/1(torque_cm) -> Merge1/1
  LCaccel_cmd/1 -> Subsystem1/1(acc_cmd)
  Merge2/1 -> BrakeCm/1
  ACCaccel_cmd/1 -> Subsystem2/1(acc_cmd)
  Merge1/1 -> TorgueCm/1
  Select/1 -> Switch Case1/1

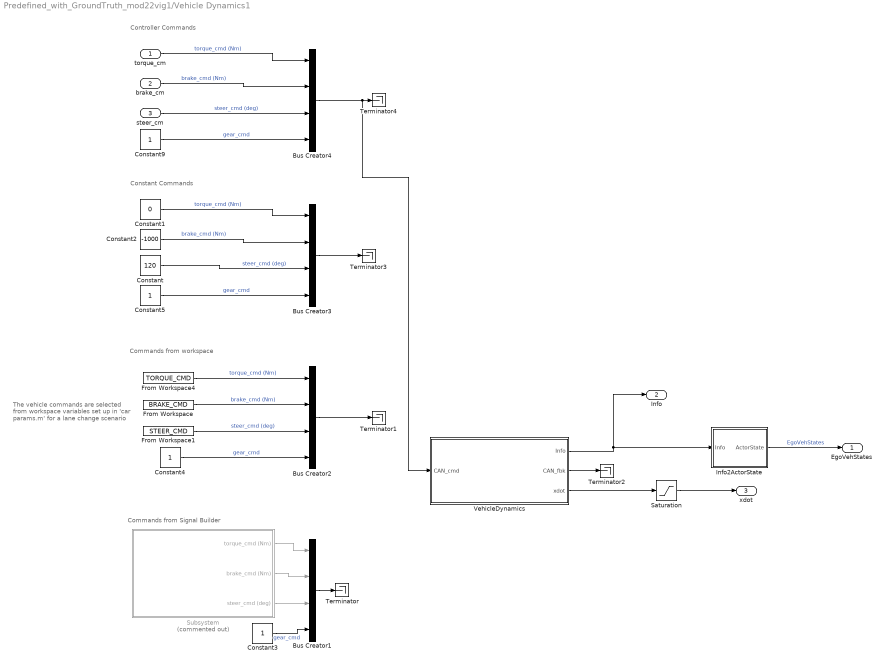
== system Predefined_with_GroundTruth_mod22vig1/Vehicle Dynamics1 ==
  note: Constant Commands
  note: Commands from workspace
  note: Commands from Signal Builder
  note: The vehicle commands are selected from workspace variables set up in 'car params.m' for a lane change scenario
  note: Controller Commands
  torque_cm : Inport
  brake_cm : Inport  Port=2
  steer_cm : Inport  Port=3
  Bus Creator{1..4} (4 alike) : BusCreator  Inputs=4
  Constant : Constant  Value=120
  Constant1 : Constant  Value=0
  Constant2 : Constant  Value=-1000
  Constant{3..5,9} (4 alike) : Constant
  From Workspace : FromWorkspace  VariableName=BRAKE_CMD  SampleTime=ts
  From Workspace1 : FromWorkspace  VariableName=STEER_CMD  SampleTime=ts
  From Workspace4 : FromWorkspace  VariableName=TORQUE_CMD  SampleTime=ts
  Info2ActorState : Subsystem
  Saturation : Saturate  UpperLimit=inf  LowerLimit=0.001
  Subsystem : Subsystem  Commented=on
  Terminator{,1..4} (5 alike) : Terminator
  VehicleDynamics : Subsystem  mask{InitPosition=[X_o Y_o 0], InitSpeed=0, InitYaw=psi_o}
      mask prompts: InitPosition "Initial Position (m)"; InitSpeed "Initial Speed (m/s)"; InitYaw "Init Yaw (rad)"
  EgoVehStates : Outport
  Info : Outport  Port=2
  xdot : Outport  Port=3
  wires:
  Bus Creator2/1 -> Terminator1/1
  VehicleDynamics/2(CAN_fbk) -> Terminator2/1
  VehicleDynamics/1(Info) -> Info/1, Info2ActorState/1(Info)
  Constant/1 -> Bus Creator3/3  "steer_cmd (deg)"
  Info2ActorState/1(ActorState) -> EgoVehStates/1  "EgoVehStates"
  Constant1/1 -> Bus Creator3/1  "torque_cmd (Nm)"
  Constant2/1 -> Bus Creator3/2  "brake_cmd (Nm)"
  VehicleDynamics/3(xdot) -> Saturation/1
  Subsystem/1(torque_cmd (Nm)) -> Bus Creator1/1
  Subsystem/2(brake_cmd (Nm)) -> Bus Creator1/2
  Subsystem/3(steer_cmd (deg)) -> Bus Creator1/3
  Constant3/1 -> Bus Creator1/4  "gear_cmd"
  Constant4/1 -> Bus Creator2/4  "gear_cmd"
  From Workspace/1 -> Bus Creator2/2  "brake_cmd (Nm)"
  From Workspace1/1 -> Bus Creator2/3  "steer_cmd (deg)"
  From Workspace4/1 -> Bus Creator2/1  "torque_cmd (Nm)"
  Constant5/1 -> Bus Creator3/4  "gear_cmd"
  Bus Creator1/1 -> Terminator/1
  brake_cm/1 -> Bus Creator4/2  "brake_cmd (Nm)"
  Constant9/1 -> Bus Creator4/4  "gear_cmd"
  torque_cm/1 -> Bus Creator4/1  "torque_cmd (Nm)"
  steer_cm/1 -> Bus Creator4/3  "steer_cmd (deg)"
  Bus Creator3/1 -> Terminator3/1
  Bus Creator4/1 -> VehicleDynamics/1(CAN_cmd), Terminator4/1
  Saturation/1 -> xdot/1

== system Predefined_with_GroundTruth_mod22vig1/Visualization ==
  note: Visualization
  TL1_poses : Inport
  Actors : Inport  Port=2
  EgoInfo : Inport  Port=3
  ss1_poses : Inport  Port=4
  Visualization : MATLABSystem  System=TL_vis
      mask Type: TL_vis
      mask Display:
      | disp('TL_vis');
      | port_label('input',1,'TL');
      | port_label('input',2,'TargetPoses');
      | port_label('input',3,'EgoInfo');
      | port_label('input',4,'SS');
  wires:
  EgoInfo/1 -> Visualization/3
  Actors/1 -> Visualization/2  "target_vehicle_poses"
  TL1_poses/1 -> Visualization/1
  ss1_poses/1 -> Visualization/4

== system Predefined_with_GroundTruth_mod22vig1/Positions and States /Traffic Light Sensor ==
  note: Traffic Light Sensor
  TL_id : Inport
  Bus Creator : BusCreator  Inputs=2
  LightConfiguration : Constant  Value=TrafficLightSensorModeSelection
  Traffic Light Switching Logic : Stateflow chart  TreatAsAtomicUnit=on
  TL_State : Outport
  wires:
  LightConfiguration/1 -> Traffic Light Switching Logic/1(LightConfig)
  TL_id/1 -> Traffic Light Switching Logic/2(TL_id)
  Bus Creator/1 -> TL_State/1
  Traffic Light Switching Logic/2(trafficLight) -> Bus Creator/1
  Traffic Light Switching Logic/1(TL_ID) -> Bus Creator/2

== system Predefined_with_GroundTruth_mod22vig1/Pure Pursuit Controller1/Wheel Steering Angle Formulation ==
  alpha : Inport
  Bicycle length : Constant  Value=L
  Constant : Constant  Value=2
  Divide : Product  Inputs=*/
  Lookahead distance : Constant  Value=ld
  Product : Product
  Product1 : Product
  Sine Wave : Sin  TimeSource=Use external signal  SampleTime=0
  Trigonometric Function : Trigonometry  Operator=atan
  Al : Outport
  wires:
  Sine Wave/1 -> Product1/2
  Bicycle length/1 -> Product/2
  Constant/1 -> Product/1
  Product1/1 -> Divide/1
  Product/1 -> Product1/1
  Divide/1 -> Trigonometric Function/1
  Trigonometric Function/1 -> Al/1
  alpha/1 -> Sine Wave/1
  Lookahead distance/1 -> Divide/2

== system Predefined_with_GroundTruth_mod22vig1/Reference Data/Theta ==
  note: 1) Add Subsystem or Model blocks as valid variant choices.
      | 2) You cannot connect blocks at this level. At simulation, connectivity is automatically
      | determined, based on the active variant and port name matching.
  y : Inport
  x : Inport  Port=2
  dis : Inport  Port=3
  thetaBlocks : Subsystem  VariantControl=thetaSimulinkBlock
  thetaLt : Subsystem  VariantControl=thetaLookUpTable
  theta : Outport
